simulink model "problem1_model_pretty"  (R2023b)
settings: Solver=ode8  StartTime=0.0  StopTime=30  FixedStep=1e-3  RelTol=1e-3
values from neighbouring files (symbols this model uses):
  Amp = Amps(i)    [plotting_from_sim.m]
  freq = Freq(j)    [plotting_from_sim.m]
  h = A_3    (= 2)    [plotting_from_sim.m]    (also in problem1.m; problem1_1.m; proj_cnl_exer_21.m = x1-x2)
  ic = 0    [plotting_from_sim.m]    (also in problem1_1.m)
  k = 2    [plotting_from_sim.m]    (also in problem1.m; problem1_1.m)
  M_2 = 1    [plotting_from_sim.m]    (also in problem1_1.m)
  M_3 = B_3    (= 0.5)    [plotting_from_sim.m]    (also in problem1_1.m)
  S_1 = A_1    (= 0.5)    [plotting_from_sim.m]    (also in problem1_1.m)
  S_2 = A_2    (= 1)    [plotting_from_sim.m]    (also in problem1_1.m)
libraries: cstblocks x3
settings Model: Creator=afons  LastModifiedBy=afons

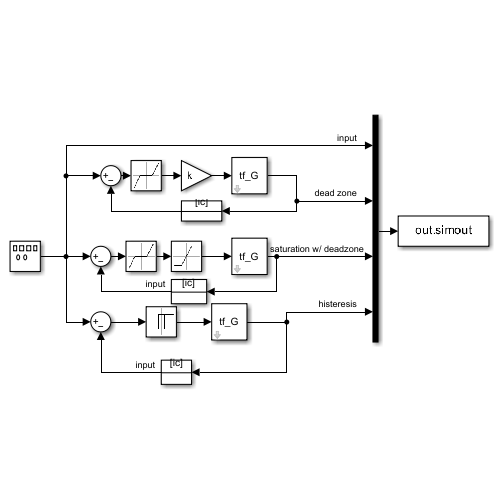
[thumbnail: Simulink's stored preview of the top-level diagram]
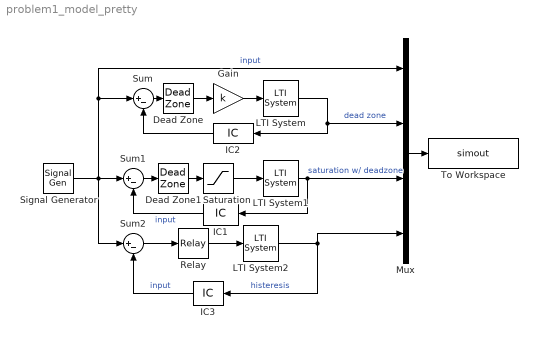
== system problem1_model_pretty ==
  Dead Zone : DeadZone  LowerValue=-S_1  UpperValue=S_1
  Dead Zone1 : DeadZone  LowerValue=-S_2  UpperValue=S_2
  Gain : Gain  Gain=k
  IC1 : InitialCondition  Value=ic
  IC2 : InitialCondition  Value=ic
  IC3 : InitialCondition  Value=ic
  LTI System : cstblocks/LTI System  sys=tf_G  IC=[]  PadeOrder=0
  LTI System1 : cstblocks/LTI System  sys=tf_G  IC=[]  PadeOrder=0
  LTI System2 : cstblocks/LTI System  sys=tf_G  IC=[]  PadeOrder=0
  Mux : Mux
  Relay : Relay  OnSwitchValue=h  OffSwitchValue=-h  OnOutputValue=M_3  OffOutputValue=-M_3
  Saturation : Saturate  UpperLimit=M_2  LowerLimit=-M_2
  Signal Generator : SignalGenerator  Amplitude=Amp  Frequency=freq  Units=rad/sec
  Sum : Sum  Inputs=|+-
  Sum1 : Sum  Inputs=|+-
  Sum2 : Sum  Inputs=|+-
  To Workspace : ToWorkspace  VariableName=simout  SaveFormat=Timeseries  SampleTime=-1
  wires:
  Dead Zone1/1 -> Saturation/1
  Sum/1 -> Dead Zone/1
  LTI System/1 -> IC2/1, Mux/2  "dead zone"
  LTI System1/1 -> IC1/1, Mux/3  "saturation w/ deadzone"
  Saturation/1 -> LTI System1/1
  Sum1/1 -> Dead Zone1/1
  LTI System2/1 -> IC3/1, Mux/4  "histeresis"
  Relay/1 -> LTI System2/1
  Sum2/1 -> Relay/1
  Dead Zone/1 -> Gain/1
  Gain/1 -> LTI System/1
  Signal Generator/1 -> Sum2/1, Sum/1, Mux/1, Sum1/1  "input"
  IC2/1 -> Sum/2
  IC1/1 -> Sum1/2  "input"
  IC3/1 -> Sum2/2  "input"
  Mux/1 -> To Workspace/1
